simulink model "ch_5_10"  (Simulink 6.3)
settings: Solver=ode45  StartTime=0.0  StopTime=10.0  RelTol=1e-3
libraries: commutil2 x2, dspquant2 x2
settings Model: LastModifiedBy=Yuantao Gu

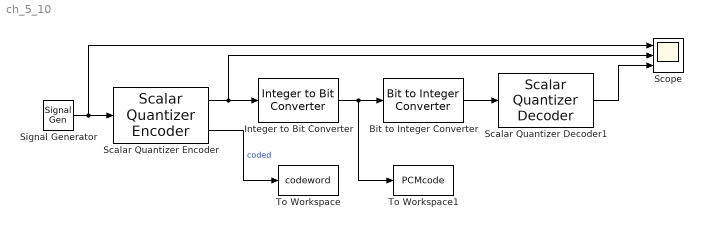
== system ch_5_10 ==
  Bit to Integer Converter : commutil2/Bit to Integer Converter  nbits=4  outDtype=Same as input
  Integer to Bit Converter : commutil2/Integer to Bit Converter  nbits=4  outDtype=Same as input
  Scalar Quantizer Decoder1 : dspquant2/Scalar Quantizer Decoder  CBsource=Specify via dialog  invalidin=Clip  codebook=[-0.9:0.2:0.9]  dataType=double  isSigned=on  wordLen=16  udDataType=sfix(16)  fracBitsMode=Best precision  numFracBits=11
  Scalar Quantizer Encoder : dspquant2/Scalar Quantizer Encoder  paramSrc=Specify via dialog  partType=Bounded  BBoundary=[-1:0.2:1]  UBoundary=[2:9]  SearchMethod=Linear  tieBreakRule=Choose the lower index  outQU=on  outQError=off  codebook=[-0.9:0.2:0.9]  outStatus=off  invalidin=Clip  idtype=int32  roundingMode=Floor  overflowMode=off
  Scope : Scope  NumInputPorts=3
      settings: YMin=-2~-2~-5  YMax=2~2~5  SampleInput=on  SampleTime=0.01
  Signal Generator : SignalGenerator  Frequency=0.1
  To Workspace : ToWorkspace  VariableName=codeword  SampleTime=1  SaveFormat=Array
  To Workspace1 : ToWorkspace  VariableName=PCMcode  SampleTime=1  SaveFormat=Array
  wires:
  Scalar Quantizer Encoder/2 -> To Workspace/1  "coded"
  Signal Generator/1 -> Scalar Quantizer Encoder/1, Scope/1
  Bit to Integer Converter/1 -> Scalar Quantizer Decoder1/1
  Scalar Quantizer Decoder1/1 -> Scope/3
  Integer to Bit Converter/1 -> Bit to Integer Converter/1, To Workspace1/1
  Scalar Quantizer Encoder/1 -> Integer to Bit Converter/1, Scope/2
